simulink model "ACC01"  (R2016b)
settings: Solver=VariableStepAuto  StartTime=0.0  StopTime=50  RelTol=1e-3
libraries: simulink x1, Solver_SF x1
settings Model: Creator=Administrator  LastModifiedBy=Administrator

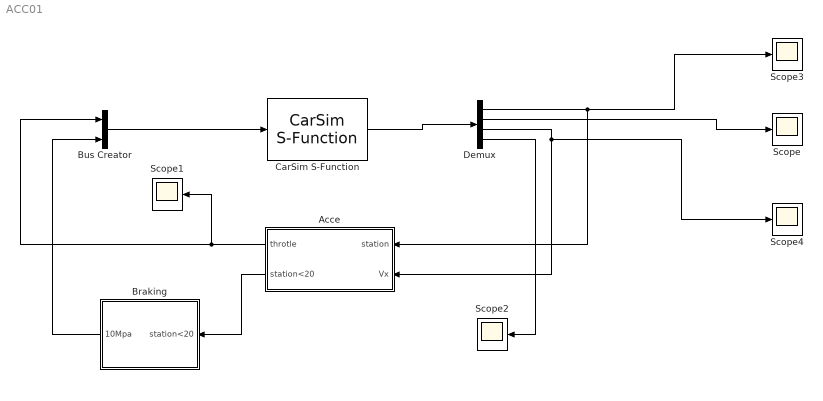
== system ACC01 ==
  Acce : Subsystem
  Braking : Subsystem
  Bus Creator : BusCreator  Inputs=2
  CarSim S-Function : Solver_SF/CarSim S-Function  Priority=1  VehicleCode=i_i  SIMFILE=Simfile.sim
  Demux : Demux
  Scope{,1..4} (5 alike) : Scope
  wires:
  CarSim S-Function/1 -> Demux/1
  Bus Creator/1 -> CarSim S-Function/1
  Demux/1 -> Acce/1(station), Scope3/1
  Acce/1(throtle) -> Bus Creator/1, Scope1/1
  Acce/2(station<20) -> Braking/1(station<20)
  Braking/1(10Mpa) -> Bus Creator/2
  Demux/2 -> Scope/1
  Demux/3 -> Scope4/1, Acce/2(Vx)
  Demux/4 -> Scope2/1

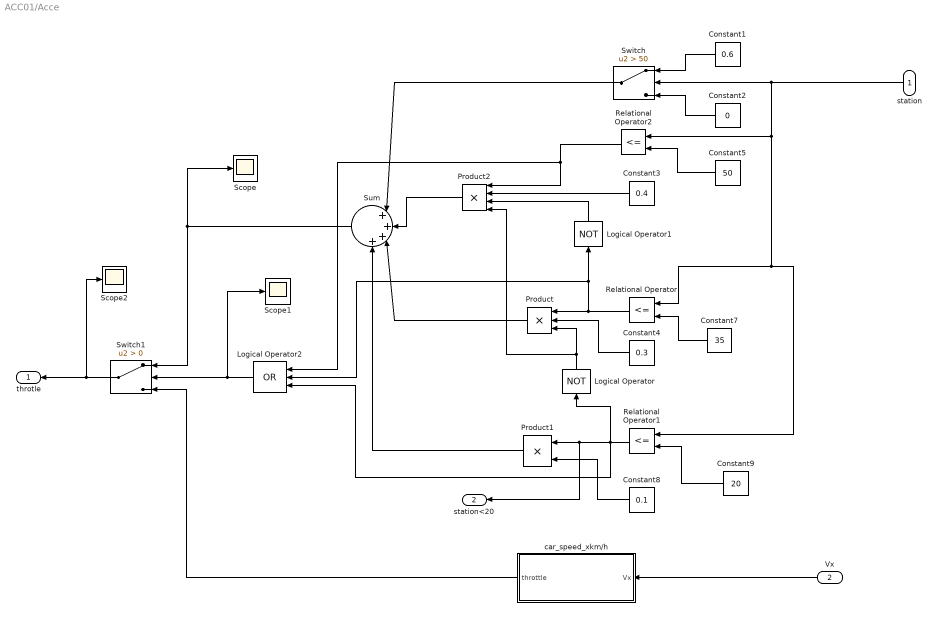
== system ACC01/Acce ==
  station : Inport
  Vx : Inport  Port=2
  Constant1 : Constant  Value=0.6
  Constant2 : Constant  Value=0
  Constant3 : Constant  Value=0.4
  Constant4 : Constant  Value=0.3
  Constant5 : Constant  Value=50
  Constant7 : Constant  Value=35
  Constant8 : Constant  Value=0.1
  Constant9 : Constant  Value=20
  Logical Operator : Logic  Operator=NOT  Inputs=1  AllPortsSameDT=off  OutDataTypeStr=boolean
  Logical Operator1 : Logic  Operator=NOT  Inputs=1  AllPortsSameDT=off  OutDataTypeStr=boolean
  Logical Operator2 : Logic  Operator=OR  Inputs=3  AllPortsSameDT=off  OutDataTypeStr=boolean
  Product : Product  Inputs=3
  Product1 : Product
  Product2 : Product  Inputs=4
  Relational Operator : RelationalOperator  Operator=<=  OutDataTypeStr=boolean  RndMeth=Simplest
  Relational Operator1 : RelationalOperator  Operator=<=  OutDataTypeStr=boolean  RndMeth=Simplest
  Relational Operator2 : RelationalOperator  Operator=<=  OutDataTypeStr=boolean  RndMeth=Simplest
  Scope : Scope
  Scope1 : Scope
  Scope2 : Scope
  Sum : Sum  Inputs=|++++
  Switch : Switch  Criteria=u2 > Threshold  Threshold=50
  Switch1 : Switch  Criteria=u2 > Threshold
  car_speed_xkm/h : Subsystem
  throtle : Outport
  station<20 : Outport  Port=2
  wires:
  station/1 -> Switch/2, Relational Operator2/1, Relational Operator1/1, Relational Operator/1
  Constant7/1 -> Relational Operator/2
  Relational Operator/1 -> Product/1, Logical Operator2/2, Logical Operator1/1
  Constant4/1 -> Product/2
  Constant9/1 -> Relational Operator1/2
  Relational Operator1/1 -> Logical Operator/1, Logical Operator2/3, station<20/1, Product1/1
  Constant8/1 -> Product1/2
  Logical Operator/1 -> Product2/4, Product/3
  Constant5/1 -> Relational Operator2/2
  Relational Operator2/1 -> Logical Operator2/1, Product2/1
  Constant3/1 -> Product2/2
  Logical Operator1/1 -> Product2/3
  Constant1/1 -> Switch/1
  Constant2/1 -> Switch/3
  Switch/1 -> Sum/1
  Product2/1 -> Sum/2
  Product/1 -> Sum/3
  Product1/1 -> Sum/4
  Vx/1 -> car_speed_xkm/h/1(Vx)
  car_speed_xkm/h/1(throttle) -> Switch1/3
  Sum/1 -> Scope/1, Switch1/1
  Logical Operator2/1 -> Scope1/1, Switch1/2
  Switch1/1 -> Scope2/1, throtle/1

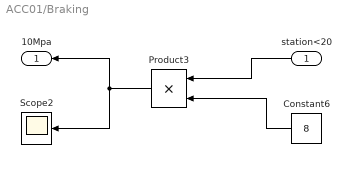
== system ACC01/Braking ==
  station<20 : Inport
  Constant6 : Constant  Value=8
  Product3 : Product
  Scope2 : Scope
  10Mpa : Outport
  wires:
  station<20/1 -> Product3/1
  Constant6/1 -> Product3/2
  Product3/1 -> 10Mpa/1, Scope2/1

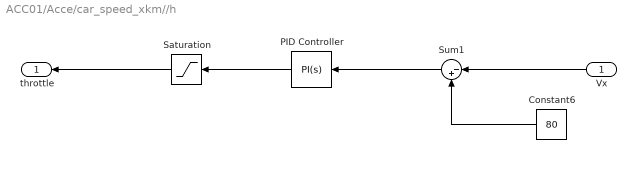
== system ACC01/Acce/car_speed_xkm//h ==
  Vx : Inport
  Constant6 : Constant  Value=80
  PID Controller : simulink/Continuous/PID Controller  Controller=PI  TimeDomain=Continuous-time  SampleTime=-1  IntegratorMethod=Forward Euler  FilterMethod=Forward Euler  Form=Parallel  UseFilter=on  ControllerParametersSource=internal  P=10  I=0.01  D=0  N=100  InitialConditionSource=internal  InitialConditionForIntegrator=0  InitialConditionForFilter=0  ExternalReset=none  LimitOutput=off  UpperSaturationLimit=inf  LowerSaturationLimit=-inf  LinearizeAsGain=on  AntiWindupMode=none  Kb=1  TrackingMode=off  Kt=1  PParamMin=[]  PParamMax=[]  IParamMin=[]  IParamMax=[]  DParamMin=[]  DParamMax=[]  NParamMin=[]  NParamMax=[]  KbParamMin=[]  KbParamMax=[]  KtParamMin=[]  KtParamMax=[]  POutMin=[]  POutMax=[]  IOutMin=[]  IOutMax=[]  DOutMin=[]  DOutMax=[]  NOutMin=[]  NOutMax=[]  KbOutMin=[]  KbOutMax=[]  KtOutMin=[]  KtOutMax=[]  IntegratorOutMin=[]  IntegratorOutMax=[]  FilterOutMin=[]  FilterOutMax=[]  SumOutMin=[]  SumOutMax=[]  SumI1OutMin=[]  SumI1OutMax=[]  SumI2OutMin=[]  SumI2OutMax=[]  SumI3OutMin=[]  SumI3OutMax=[]  SumDOutMin=[]  SumDOutMax=[]  SaturationOutMin=[]  SaturationOutMax=[]  IntegratorContinuousStateAttributes=''  IntegratorStateMustResolveToSignalObject=off  IntegratorRTWStateStorageClass=Auto  FilterContinuousStateAttributes=''  FilterStateMustResolveToSignalObject=off  FilterRTWStateStorageClass=Auto  DifferentiatorICPrevScaledInput=0  DifferentiatorOutMin=[]  DifferentiatorOutMax=[]
  Saturation : Saturate  UpperLimit=1  LowerLimit=0
  Sum1 : Sum  Inputs=|-+
  throttle : Outport
  wires:
  Saturation/1 -> throttle/1
  PID Controller/1 -> Saturation/1
  Sum1/1 -> PID Controller/1
  Constant6/1 -> Sum1/2
  Vx/1 -> Sum1/1
